simulink model "ex9slidingimp"  (R2025b)
settings: Solver=VariableStepAuto  StartTime=0.0  StopTime=100  RelTol=1e-3
settings Model: Creator=Esteban  LastModifiedBy=Esteban

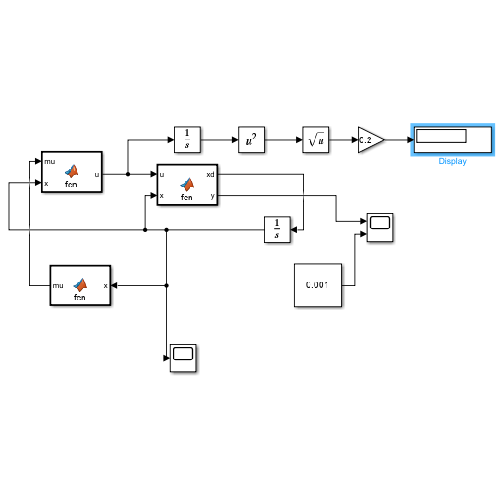
[thumbnail: Simulink's stored preview of the top-level diagram]
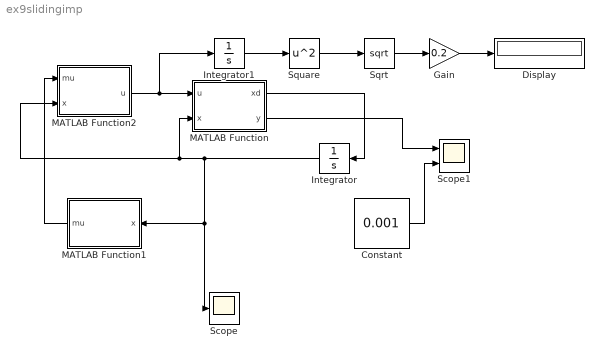
== system ex9slidingimp ==
  Constant : Constant  Value=0.001
  Display : Display
  Gain : Gain  Gain=0.2
  Integrator : Integrator  InitialCondition=[-7/2;4]
  Integrator1 : Integrator
  MATLAB Function : MATLAB Function  TreatAsAtomicUnit=on
  MATLAB Function1 : MATLAB Function  TreatAsAtomicUnit=on
  MATLAB Function2 : MATLAB Function  TreatAsAtomicUnit=on
  Scope : Scope
  Scope1 : Scope  NumInputPorts=2
  Sqrt : Sqrt
  Square : Math  Operator=square
  wires:
  MATLAB Function/1(xd) -> Integrator/1
  Integrator/1 -> Scope/1, MATLAB Function1/1(x), MATLAB Function2/2(x), MATLAB Function/2(x)
  MATLAB Function2/1(u) -> Integrator1/1, MATLAB Function/1(u)
  MATLAB Function1/1(mu) -> MATLAB Function2/1(mu)
  Integrator1/1 -> Square/1
  Square/1 -> Sqrt/1
  Sqrt/1 -> Gain/1
  Constant/1 -> Scope1/2
  MATLAB Function/2(y) -> Scope1/1
  Gain/1 -> Display/1

== matlab function ex9slidingimp/MATLAB Function ==
  data: u input; xd output; x input; y output
function [xd,y] = fcn(u,x)

xd = [x(2);
    -0.2*x(1)^3+x(1)-u-3*x(2)];

y = x(1);

== matlab function ex9slidingimp/MATLAB Function2 ==
  data: mu input; u output; x input
function u = fcn(mu, x)

eta = 1;
k1 = 9;
k2 = 9;
s = mu(2) + k2*mu(1);
v = -k2*mu(1) -k1*tanh(s*eta);
u = -x(1)^3/5 + x(1) - v - 3*x(2);

== matlab function ex9slidingimp/MATLAB Function1 ==
  data: x input; mu output
function mu = fcn(x)

mu = [x(1);x(2)];
